simulink model "Pitch_Equation_Model"  (R2023b)
settings: Solver=VariableStepAuto  StartTime=0.0  StopTime=10.0  RelTol=1e-3
libraries: shareddyn x1, ctrlSharedLib x1, aerolibbdyn x1
settings Model: Creator=ricca  LastModifiedBy=ricca

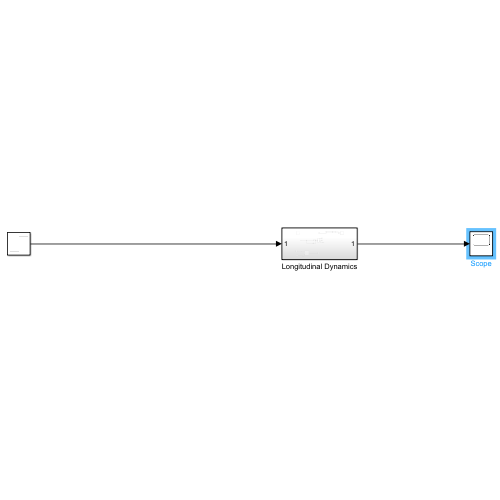
[thumbnail: Simulink's stored preview of the top-level diagram]
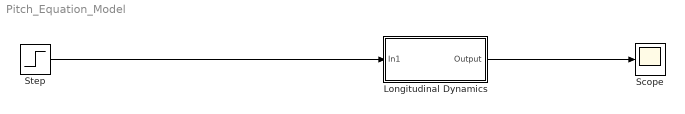
== system Pitch_Equation_Model ==
  Longitudinal Dynamics : Subsystem
  Scope : Scope
  Step : Step  SampleTime=0
  wires:
  Longitudinal Dynamics/1(Output) -> Scope/1
  Step/1 -> Longitudinal Dynamics/1(In1)

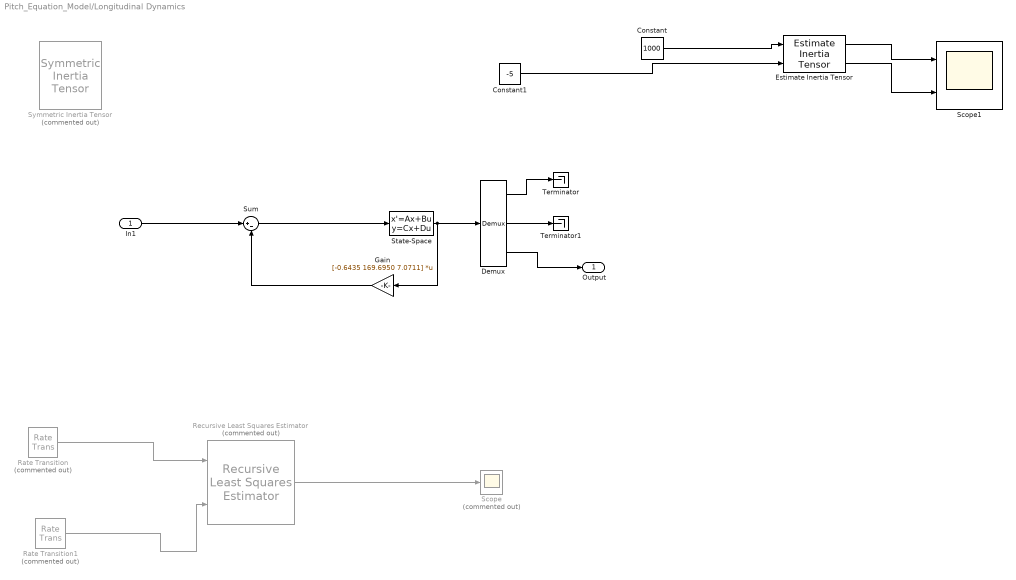
== system Pitch_Equation_Model/Longitudinal Dynamics ==
  In1 : Inport
  Constant : Constant  Value=1000
  Constant1 : Constant  Value=-5
  Demux : Demux  Outputs=3
  Estimate Inertia Tensor : shareddyn/Estimate Inertia Tensor  fmass=2  emass=1  fI=eye(3)  eI=eye(3)/2  aMode=aMode
      settings: LibrarySourceBlock=|
      | aerolibbdyn/Estimate
      | Inertia Tensor
  Gain : Gain  Gain=[-0.6435 169.6950 7.0711]  Multiplication=Matrix(K*u)
  Rate Transition : RateTransition  Commented=on
  Rate Transition1 : RateTransition  Commented=on
  Recursive Least Squares Estimator : ctrlSharedLib/Recursive Least Squares Estimator  Commented=on  InitialEstimateSource=None  InitialParameterData=1  P0=1e4  InitialRegressors=0  InitialOutputs=0  History=Infinite  WindowLength=200  EstimationMethod=Forgetting Factor  AdaptationParameter=1  HasTimeVaryingAdaptationParameter=off  NormalizationBias=eps  OutputError=off  OutputP=off  AddEnablePort=off  InputProcessing=Sample-based  Ts=-1
      settings: LibrarySourceBlock=slident/Estimators/Recursive Least Squares Estimator
  Scope : Scope  Commented=on
  Scope1 : Scope  NumInputPorts=2
  State-Space : StateSpace  A=[-0.313 56.7 0; -0.0139 -0.426 0; 0 56.7 0]  B=[0.232; 0.0203; 0]  C=eye(3)  D=[0;0;0]  InitialCondition=0
  Sum : Sum  Inputs=|+-
  Symmetric Inertia Tensor : aerolibbdyn/Symmetric Inertia Tensor  Commented=on
  Terminator : Terminator
  Terminator1 : Terminator
  Output : Outport
  wires:
  Recursive Least Squares Estimator/1 -> Scope/1
  Constant/1 -> Estimate Inertia Tensor/1
  Estimate Inertia Tensor/1 -> Scope1/1
  Estimate Inertia Tensor/2 -> Scope1/2
  Constant1/1 -> Estimate Inertia Tensor/2
  Rate Transition/1 -> Recursive Least Squares Estimator/1
  Rate Transition1/1 -> Recursive Least Squares Estimator/2
  State-Space/1 -> Gain/1, Demux/1
  Demux/1 -> Terminator/1
  Demux/3 -> Output/1
  Demux/2 -> Terminator1/1
  In1/1 -> Sum/1
  Sum/1 -> State-Space/1
  Gain/1 -> Sum/2
